simulink model "StirringTankHeater"  (R2023a)
settings: Solver=VariableStepAuto  StartTime=0.0  StopTime=20  FixedStep=0.0000001  RelTol=1e-3
libraries: simulink x1
settings Model: Creator=intel  LastModifiedBy=intel

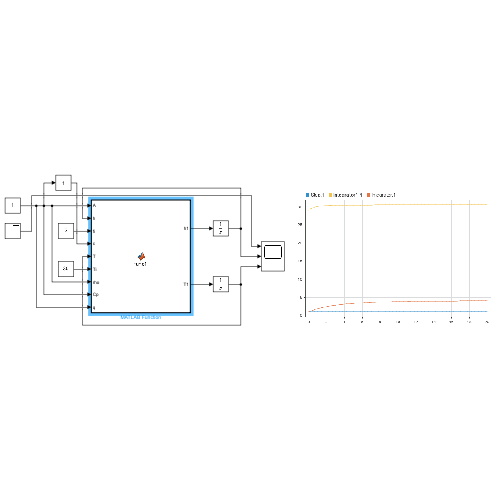
[thumbnail: Simulink's stored preview of the top-level diagram]
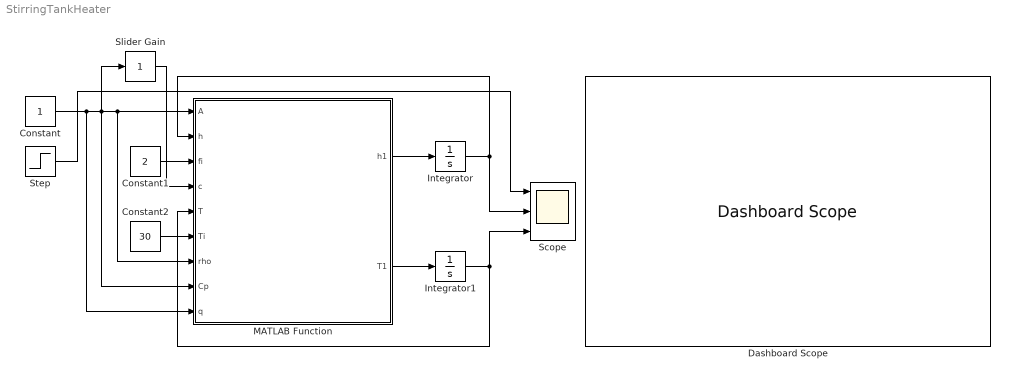
== system StirringTankHeater ==
  Constant : Constant
  Constant1 : Constant  Value=2
  Constant2 : Constant  Value=30
  Dashboard Scope : DashboardScope
  Integrator : Integrator  InitialCondition=1
  Integrator1 : Integrator  InitialCondition=29
  MATLAB Function : MATLAB Function  TreatAsAtomicUnit=on
  Scope : Scope  NumInputPorts=3
  Slider Gain : simulink/Math Operations/Slider Gain  gain=1  low=0  high=2
  Step : Step  Time=0  SampleTime=0
  wires:
  Step/1 -> Scope/1
  Constant/1 -> MATLAB Function/9(q), MATLAB Function/1(A), MATLAB Function/7(rho), Slider Gain/1, MATLAB Function/8(Cp)
  MATLAB Function/1(h1) -> Integrator/1
  MATLAB Function/2(T1) -> Integrator1/1
  Integrator1/1 -> MATLAB Function/5(T), Scope/3
  Integrator/1 -> Scope/2, MATLAB Function/2(h)
  Slider Gain/1 -> MATLAB Function/4(c)
  Constant1/1 -> MATLAB Function/3(fi)
  Constant2/1 -> MATLAB Function/6(Ti)

== matlab function StirringTankHeater/MATLAB Function ==
  data: A input; h1 output; h input; fi input; c input; T input; Ti input; rho input; Cp input; q input; T1 output
function [h1, T1] = func1(A, h, fi, c, T, Ti, rho, Cp, q)

h1 = (fi - c*sqrt(h))/A;
T1 = ((fi*(Ti-T)) + q/(rho*Cp))/(A*h);
